simulink model "Touch_identifier"  (R2017b)
settings: Solver=VariableStepAuto  StartTime=0.0  StopTime=10.0  RelTol=1e-3
settings Model: Creator=Kalana  LastModifiedBy=Kalana

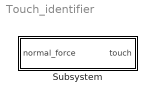
== system Touch_identifier ==
  Subsystem : Subsystem

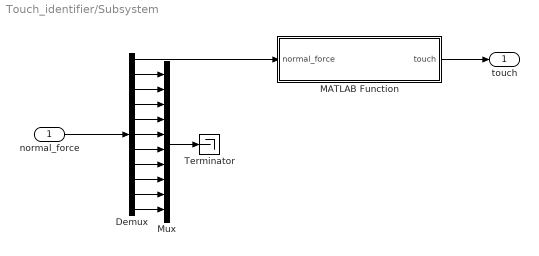
== system Touch_identifier/Subsystem ==
  normal_force : Inport
  Demux : Demux  Outputs=11
  MATLAB Function : MATLAB Function  TreatAsAtomicUnit=on
  Mux : Mux  Inputs=10
  Terminator : Terminator
  "touch " : Outport
  wires:
  Demux/10 -> Mux/9
  Demux/7 -> Mux/6
  Demux/6 -> Mux/5
  MATLAB Function/1(touch) -> "touch "/1
  Demux/11 -> Mux/10
  Demux/3 -> Mux/2
  Demux/4 -> Mux/3
  Demux/8 -> Mux/7
  Mux/1 -> Terminator/1
  Demux/5 -> Mux/4
  normal_force/1 -> Demux/1
  Demux/9 -> Mux/8
  Demux/2 -> Mux/1
  Demux/1 -> MATLAB Function/1(normal_force)

== matlab function Touch_identifier/Subsystem/MATLAB Function ==
  data: normal_force input; touch output
function touch = TouchIdentifier(normal_force)

if normal_force>0
    touch = 1;
else
    touch = 0;
end
